simulink model "Sim_V_in"  (R2024b)
settings: Solver=VariableStepAuto  StartTime=0  StopTime=sim.t  RelTol=1e-6  AbsTol=1e-6
undefined symbols (not defined in the file or in its folder): cube, Earth, h, motor, sim, WGS84
libraries: slpidlib x3, aerolibfltsims x2, aerolibtransform2 x1, aerolibanim x1
settings Model: Creator=ben  LastModifiedBy=ben
settings DataIOCC: SaveFormat=StructureWithTime
settings OptimizationCC: BlockReduction=off  BufferReuse=off
settings DebuggingCC: SignalInfNanChecking=warning  AlgebraicLoopMsg=none  CheckMatrixSingularityMsg=warning  UnderSpecifiedDataTypeMsg=warning  UnderSpecifiedDimensionMsg=warning

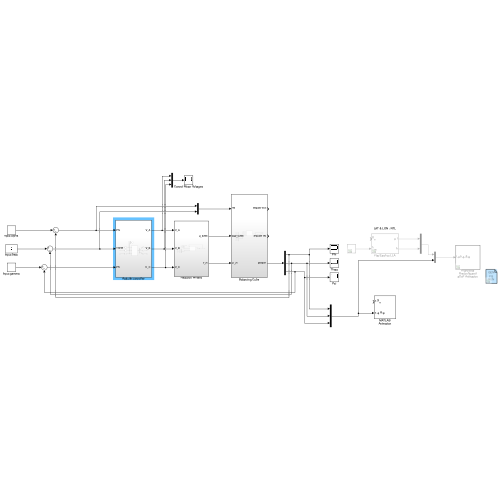
[thumbnail: Simulink's stored preview of the top-level diagram]
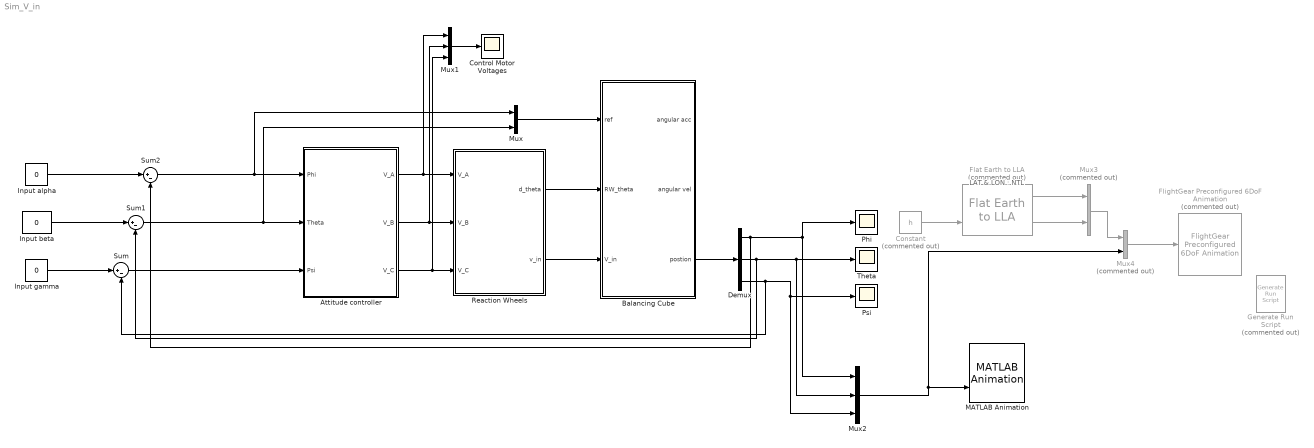
== system Sim_V_in ==
  note: LAT & LON : NTL
  Attitude controller : Subsystem
  Balancing Cube : Subsystem
  Constant : Constant  Commented=on  Value=h
  Control Motor Voltages : Scope
  Demux : Demux  Outputs=3
  Flat Earth to LLA : aerolibtransform2/Flat Earth to LLA  Commented=on  units=Metric (MKS)  ptype=Earth (WGS84)  F=1/298.257223563  R=6378137  refPosPort=off  LL0=[22 150]  psi=0
  FlightGear Preconfigured 6DoF Animation : aerolibfltsims/FlightGear Preconfigured 6DoF Animation  Commented=on  xFlightGearVersion=v2019.1  DestinationIpAddress=127.0.0.1  DestinationPort=5502  SampleTime=1/20  packetVersion=24
  Generate Run Script : aerolibfltsims/Generate Run Script  Commented=on  Architecture=Mac  dataFlow=Send  GeometryModelName=c172p  AirportId=YSSY  RunwayId=10L  InitialAltitude=7224  InitialHeading=113  OffsetDistance=4.72  OffsetAzimuth=0  InstallScenery=on  DisableShaders=on  OriginAddress=127.0.0.1  DestinationPort=5502  OriginPort=5505  LocalAddress=127.0.0.1  OutputFileName=runfg2.sh  FlightGearBaseDirectory=/Applications/FlightGear.app
  Input alpha : Constant  Value=0  SampleTime=0.1
  Input beta : Constant  Value=0  SampleTime=0.1
  Input gamma : Constant  Value=0  SampleTime=0.1
  MATLAB Animation : aerolibanim/MATLAB Animation  Tag=Matlab Animation 6 DOF  Vehicles=1  Geometries='pa24-250_orange.ac'  BoundingBoxCoordinates=[-50,50,-50,50,-50,50]  CameraOffset=[-150,0,0]  CameraViewAngle=5  SampleTime=0.01  FigurePosition=[761,103,744,778]
  Mux : Mux  Inputs=2
  Mux1 : Mux  Inputs=3
  Mux2 : Mux  Inputs=3
  Mux3 : Mux  Commented=on  Inputs=2
  Mux4 : Mux  Commented=on  Inputs=2
  Phi : Scope
  Psi : Scope
  Reaction Wheels : Subsystem
  Sum : Sum  Inputs=|+-
  Sum1 : Sum  Inputs=|+-
  Sum2 : Sum  Inputs=|+-
  Theta : Scope
  wires:
  Sum2/1 -> Mux/1, Attitude controller/1(Phi)
  Sum1/1 -> Attitude controller/2(Theta), Mux/2
  Sum/1 -> Attitude controller/3(Psi)
  Demux/1 -> Mux2/1, Phi/1, Sum2/2
  Demux/2 -> Mux2/2, Theta/1, Sum1/2
  Demux/3 -> Sum/2, Mux2/3, Psi/1
  Mux1/1 -> Control Motor Voltages/1
  Mux4/1 -> FlightGear Preconfigured 6DoF Animation/1
  Mux3/1 -> Mux4/1
  Mux2/1 -> MATLAB Animation/2, Mux4/2
  Flat Earth to LLA/2 -> Mux3/2
  Constant/1 -> Flat Earth to LLA/2
  Flat Earth to LLA/1 -> Mux3/1
  Input beta/1 -> Sum1/1
  Input gamma/1 -> Sum/1
  Reaction Wheels/2(v_in) -> Balancing Cube/3(V_in)
  Mux/1 -> Balancing Cube/1(ref)
  Balancing Cube/3(postion) -> Demux/1
  Input alpha/1 -> Sum2/1
  Attitude controller/1(V_A) -> Mux1/1, Reaction Wheels/1(V_A)
  Attitude controller/2(V_B) -> Mux1/2, Reaction Wheels/2(V_B)
  Attitude controller/3(V_C) -> Mux1/3, Reaction Wheels/3(V_C)
  Reaction Wheels/1(d_theta) -> Balancing Cube/2(RW_theta)

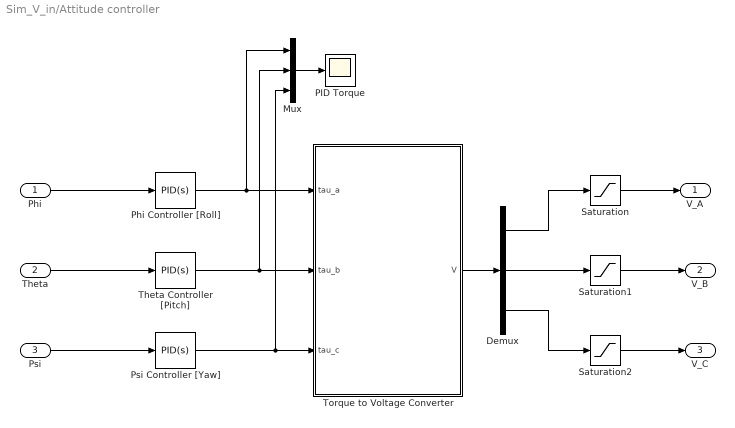
== system Sim_V_in/Attitude controller ==
  Phi : Inport
  Theta : Inport  Port=2
  Psi : Inport  Port=3
  Demux : Demux  Outputs=3
  Mux : Mux  Inputs=3
  PID Torque : Scope
  Phi Controller [Roll] : slpidlib/PID Controller  Controller=PID  Form=Parallel  TimeDomain=Continuous-time  UseExternalTs=off  SampleTime=-1  IntegratorMethod=Forward Euler  FilterMethod=Forward Euler  ControllerParametersSource=internal  P=-2.44415331656195e+90  I=-4.38149470446761e+91  UseKiTs=off  D=-3.03389489553192e+88  UseExternalDerivativeSource=off  N=5793.03682854453  UseFilter=on  TunerSelectOption=Transfer Function Based (PID Tuner App)  InitialConditionSource=internal  InitialConditionForIntegrator=0  InitialConditionForFilter=0  DifferentiatorICPrevScaledInput=0  ExternalReset=none  TrackingMode=off  Kt=1  LimitOutput=off  SatLimitsSource=internal  UpperSaturationLimit=inf  LowerSaturationLimit=-inf  LinearizeAsGain=on  AntiWindupMode=none  Kb=1  LimitIntegrator=off  UpperIntegratorSaturationLimit=inf  LowerIntegratorSaturationLimit=-inf  POutMin=[]  POutMax=[]  IOutMin=[]  IOutMax=[]  DOutMin=[]  DOutMax=[]  NOutMin=[]  NOutMax=[]  SumOutMin=[]  SumOutMax=[]  SaturationOutMin=[]  SaturationOutMax=[]  PParamMin=[]  PParamMax=[]  IParamMin=[]  IParamMax=[]  DParamMin=[]  DParamMax=[]  NParamMin=[]  NParamMax=[]  KbParamMin=[]  KbParamMax=[]  KtParamMin=[]  KtParamMax=[]  KbOutMin=[]  KbOutMax=[]  KtOutMin=[]  KtOutMax=[]  IntegratorOutMin=[]  IntegratorOutMax=[]  FilterOutMin=[]  FilterOutMax=[]  SumI1OutMin=[]  SumI1OutMax=[]  SumI2OutMin=[]  SumI2OutMax=[]  SumI3OutMin=[]  SumI3OutMax=[]  SumI4OutMin=[]  SumI4OutMax=[]  SumDOutMin=[]  SumDOutMax=[]  DifferentiatorOutMin=[]  DifferentiatorOutMax=[]  FilterDiffOutCoefMin=[]  FilterDiffOutCoefMax=[]  ReciprocalOutMin=[]  ReciprocalOutMax=[]  SumDenOutMin=[]  SumDenOutMax=[]  SumNumOutMin=[]  SumNumOutMax=[]  DivideOutMin=[]  DivideOutMax=[]  UdiffTsProdOutMin=[]  UdiffTsProdOutMax=[]  NTsProdOutMin=[]  NTsProdOutMax=[]  UintegralTsProdOutMin=[]  UintegralTsProdOutMax=[]  UngainTsProdOutMin=[]  UngainTsProdOutMax=[]  ClampingZeroOutDataTypeStr=Inherit: Inherit via back propagation  ClampingZeroOutMin=[]  ClampingZeroOutMax=[]  FilterDenConstantOutDataTypeStr=Inherit: Inherit via back propagation  FilterDenConstantOutMin=[]  FilterDenConstantOutMax=[]  PCopyOutDataTypeStr=Inherit: Inherit via back propagation  PCopyOutMin=[]  PCopyOutMax=[]  NCopyOutDataTypeStr=Inherit: Inherit via back propagation  NCopyOutMin=[]  NCopyOutMax=[]  IntegratorContinuousStateAttributes=''  IntegratorStateMustResolveToSignalObject=off  IntegratorRTWStateStorageClass=Auto  FilterContinuousStateAttributes=''  FilterStateMustResolveToSignalObject=off  FilterRTWStateStorageClass=Auto  ParallelPVariant=InternalParameters  IdealPVariant=Disabled  IVariant=InternalParameters  DVariant=InternalParameters  IntegratorVariant=Continuous  SatVariant=Disabled  AWVariant=Passthrough  PCopyVariant=Disabled  TRVariant=Disabled  FdbkBlocksVariant=Forward  IdealPFdbkVariant=Disabled  SatFdbkVariant=Disabled  DerivativeFilterVariant=ContFilter  NVariant=InternalParameters  NCopyVariant=Disabled  FilterICVariant=InternalICsFilter  IntegratorICVariant=InternalICs  ExternalResetVariant=Disabled  TRSumVariant=Passthrough  SumFdbkVariant=Disabled  SumVariant=Sum_PID  TsampFilterVariant=InternalTs  TsampNgainVariant=Passthrough  TsampIntegralVariant=Disabled_SignalSpec  ExternalSaturationOutDataTypeStr=Inherit: Same as second input  DerivativeSourceVariant=ErrorSignal  PreIntVariant=InternalPreInt
  Psi Controller [Yaw] : slpidlib/PID Controller  Controller=PID  Form=Parallel  TimeDomain=Continuous-time  UseExternalTs=off  SampleTime=-1  IntegratorMethod=Forward Euler  FilterMethod=Forward Euler  ControllerParametersSource=internal  P=-763.325878025154  I=-72.3330718489805  UseKiTs=off  D=-1552.13165448844  UseExternalDerivativeSource=off  N=226.089930864036  UseFilter=on  TunerSelectOption=Transfer Function Based (PID Tuner App)  InitialConditionSource=internal  InitialConditionForIntegrator=0  InitialConditionForFilter=0  DifferentiatorICPrevScaledInput=0  ExternalReset=none  TrackingMode=off  Kt=1  LimitOutput=off  SatLimitsSource=internal  UpperSaturationLimit=inf  LowerSaturationLimit=-inf  LinearizeAsGain=on  AntiWindupMode=none  Kb=1  LimitIntegrator=off  UpperIntegratorSaturationLimit=inf  LowerIntegratorSaturationLimit=-inf  POutMin=[]  POutMax=[]  IOutMin=[]  IOutMax=[]  DOutMin=[]  DOutMax=[]  NOutMin=[]  NOutMax=[]  SumOutMin=[]  SumOutMax=[]  SaturationOutMin=[]  SaturationOutMax=[]  PParamMin=[]  PParamMax=[]  IParamMin=[]  IParamMax=[]  DParamMin=[]  DParamMax=[]  NParamMin=[]  NParamMax=[]  KbParamMin=[]  KbParamMax=[]  KtParamMin=[]  KtParamMax=[]  KbOutMin=[]  KbOutMax=[]  KtOutMin=[]  KtOutMax=[]  IntegratorOutMin=[]  IntegratorOutMax=[]  FilterOutMin=[]  FilterOutMax=[]  SumI1OutMin=[]  SumI1OutMax=[]  SumI2OutMin=[]  SumI2OutMax=[]  SumI3OutMin=[]  SumI3OutMax=[]  SumI4OutMin=[]  SumI4OutMax=[]  SumDOutMin=[]  SumDOutMax=[]  DifferentiatorOutMin=[]  DifferentiatorOutMax=[]  FilterDiffOutCoefMin=[]  FilterDiffOutCoefMax=[]  ReciprocalOutMin=[]  ReciprocalOutMax=[]  SumDenOutMin=[]  SumDenOutMax=[]  SumNumOutMin=[]  SumNumOutMax=[]  DivideOutMin=[]  DivideOutMax=[]  UdiffTsProdOutMin=[]  UdiffTsProdOutMax=[]  NTsProdOutMin=[]  NTsProdOutMax=[]  UintegralTsProdOutMin=[]  UintegralTsProdOutMax=[]  UngainTsProdOutMin=[]  UngainTsProdOutMax=[]  ClampingZeroOutDataTypeStr=Inherit: Inherit via back propagation  ClampingZeroOutMin=[]  ClampingZeroOutMax=[]  FilterDenConstantOutDataTypeStr=Inherit: Inherit via back propagation  FilterDenConstantOutMin=[]  FilterDenConstantOutMax=[]  PCopyOutDataTypeStr=Inherit: Inherit via back propagation  PCopyOutMin=[]  PCopyOutMax=[]  NCopyOutDataTypeStr=Inherit: Inherit via back propagation  NCopyOutMin=[]  NCopyOutMax=[]  IntegratorContinuousStateAttributes=''  IntegratorStateMustResolveToSignalObject=off  IntegratorRTWStateStorageClass=Auto  FilterContinuousStateAttributes=''  FilterStateMustResolveToSignalObject=off  FilterRTWStateStorageClass=Auto  ParallelPVariant=InternalParameters  IdealPVariant=Disabled  IVariant=InternalParameters  DVariant=InternalParameters  IntegratorVariant=Continuous  SatVariant=Disabled  AWVariant=Passthrough  PCopyVariant=Disabled  TRVariant=Disabled  FdbkBlocksVariant=Forward  IdealPFdbkVariant=Disabled  SatFdbkVariant=Disabled  DerivativeFilterVariant=ContFilter  NVariant=InternalParameters  NCopyVariant=Disabled  FilterICVariant=InternalICsFilter  IntegratorICVariant=InternalICs  ExternalResetVariant=Disabled  TRSumVariant=Passthrough  SumFdbkVariant=Disabled  SumVariant=Sum_PID  TsampFilterVariant=InternalTs  TsampNgainVariant=Passthrough  TsampIntegralVariant=Disabled_SignalSpec  ExternalSaturationOutDataTypeStr=Inherit: Same as second input  DerivativeSourceVariant=ErrorSignal  PreIntVariant=InternalPreInt
  Saturation : Saturate  UpperLimit=10  LowerLimit=-10
  Saturation1 : Saturate  UpperLimit=10  LowerLimit=-10
  Saturation2 : Saturate  UpperLimit=10  LowerLimit=-10
  Theta Controller [Pitch] : slpidlib/PID Controller  Controller=PID  Form=Parallel  TimeDomain=Continuous-time  UseExternalTs=off  SampleTime=-1  IntegratorMethod=Forward Euler  FilterMethod=Forward Euler  ControllerParametersSource=internal  P=-8.13203404050408e+20  I=-3.59982541336858e+22  UseKiTs=off  D=-4.51084621020332e+18  UseExternalDerivativeSource=off  N=4975.57673271944  UseFilter=on  TunerSelectOption=Transfer Function Based (PID Tuner App)  InitialConditionSource=internal  InitialConditionForIntegrator=0  InitialConditionForFilter=0  DifferentiatorICPrevScaledInput=0  ExternalReset=none  TrackingMode=off  Kt=1  LimitOutput=off  SatLimitsSource=internal  UpperSaturationLimit=inf  LowerSaturationLimit=-inf  LinearizeAsGain=on  AntiWindupMode=none  Kb=1  LimitIntegrator=off  UpperIntegratorSaturationLimit=inf  LowerIntegratorSaturationLimit=-inf  POutMin=[]  POutMax=[]  IOutMin=[]  IOutMax=[]  DOutMin=[]  DOutMax=[]  NOutMin=[]  NOutMax=[]  SumOutMin=[]  SumOutMax=[]  SaturationOutMin=[]  SaturationOutMax=[]  PParamMin=[]  PParamMax=[]  IParamMin=[]  IParamMax=[]  DParamMin=[]  DParamMax=[]  NParamMin=[]  NParamMax=[]  KbParamMin=[]  KbParamMax=[]  KtParamMin=[]  KtParamMax=[]  KbOutMin=[]  KbOutMax=[]  KtOutMin=[]  KtOutMax=[]  IntegratorOutMin=[]  IntegratorOutMax=[]  FilterOutMin=[]  FilterOutMax=[]  SumI1OutMin=[]  SumI1OutMax=[]  SumI2OutMin=[]  SumI2OutMax=[]  SumI3OutMin=[]  SumI3OutMax=[]  SumI4OutMin=[]  SumI4OutMax=[]  SumDOutMin=[]  SumDOutMax=[]  DifferentiatorOutMin=[]  DifferentiatorOutMax=[]  FilterDiffOutCoefMin=[]  FilterDiffOutCoefMax=[]  ReciprocalOutMin=[]  ReciprocalOutMax=[]  SumDenOutMin=[]  SumDenOutMax=[]  SumNumOutMin=[]  SumNumOutMax=[]  DivideOutMin=[]  DivideOutMax=[]  UdiffTsProdOutMin=[]  UdiffTsProdOutMax=[]  NTsProdOutMin=[]  NTsProdOutMax=[]  UintegralTsProdOutMin=[]  UintegralTsProdOutMax=[]  UngainTsProdOutMin=[]  UngainTsProdOutMax=[]  ClampingZeroOutDataTypeStr=Inherit: Inherit via back propagation  ClampingZeroOutMin=[]  ClampingZeroOutMax=[]  FilterDenConstantOutDataTypeStr=Inherit: Inherit via back propagation  FilterDenConstantOutMin=[]  FilterDenConstantOutMax=[]  PCopyOutDataTypeStr=Inherit: Inherit via back propagation  PCopyOutMin=[]  PCopyOutMax=[]  NCopyOutDataTypeStr=Inherit: Inherit via back propagation  NCopyOutMin=[]  NCopyOutMax=[]  IntegratorContinuousStateAttributes=''  IntegratorStateMustResolveToSignalObject=off  IntegratorRTWStateStorageClass=Auto  FilterContinuousStateAttributes=''  FilterStateMustResolveToSignalObject=off  FilterRTWStateStorageClass=Auto  ParallelPVariant=InternalParameters  IdealPVariant=Disabled  IVariant=InternalParameters  DVariant=InternalParameters  IntegratorVariant=Continuous  SatVariant=Disabled  AWVariant=Passthrough  PCopyVariant=Disabled  TRVariant=Disabled  FdbkBlocksVariant=Forward  IdealPFdbkVariant=Disabled  SatFdbkVariant=Disabled  DerivativeFilterVariant=ContFilter  NVariant=InternalParameters  NCopyVariant=Disabled  FilterICVariant=InternalICsFilter  IntegratorICVariant=InternalICs  ExternalResetVariant=Disabled  TRSumVariant=Passthrough  SumFdbkVariant=Disabled  SumVariant=Sum_PID  TsampFilterVariant=InternalTs  TsampNgainVariant=Passthrough  TsampIntegralVariant=Disabled_SignalSpec  ExternalSaturationOutDataTypeStr=Inherit: Same as second input  DerivativeSourceVariant=ErrorSignal  PreIntVariant=InternalPreInt
  Torque to Voltage Converter : MATLAB Function  TreatAsAtomicUnit=on
  V_A : Outport
  V_B : Outport  Port=2
  V_C : Outport  Port=3
  wires:
  Phi/1 -> Phi Controller [Roll]/1
  Theta/1 -> Theta Controller [Pitch]/1
  Psi/1 -> Psi Controller [Yaw]/1
  Theta Controller [Pitch]/1 -> Mux/2, Torque to Voltage Converter/2(tau_b)
  Phi Controller [Roll]/1 -> Mux/1, Torque to Voltage Converter/1(tau_a)
  Psi Controller [Yaw]/1 -> Mux/3, Torque to Voltage Converter/3(tau_c)
  Demux/2 -> Saturation1/1
  Demux/3 -> Saturation2/1
  Mux/1 -> PID Torque/1
  Saturation/1 -> V_A/1
  Saturation1/1 -> V_B/1
  Saturation2/1 -> V_C/1
  Torque to Voltage Converter/1(V) -> Demux/1
  Demux/1 -> Saturation/1

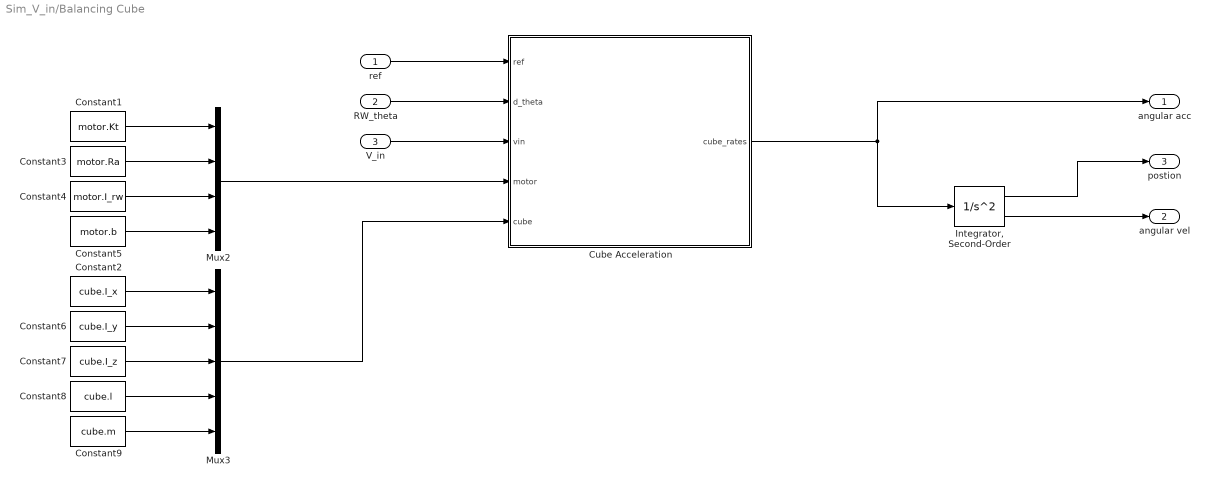
== system Sim_V_in/Balancing Cube ==
  ref : Inport
  RW_theta : Inport  Port=2
  V_in : Inport  Port=3
  Constant1 : Constant  Value=motor.Kt
  Constant2 : Constant  Value=cube.I_x
  Constant3 : Constant  Value=motor.Ra
  Constant4 : Constant  Value=motor.I_rw
  Constant5 : Constant  Value=motor.b
  Constant6 : Constant  Value=cube.I_y
  Constant7 : Constant  Value=cube.I_z
  Constant8 : Constant  Value=cube.l
  Constant9 : Constant  Value=cube.m
  Cube Acceleration : MATLAB Function  TreatAsAtomicUnit=on
  "Integrator, Second-Order" : SecondOrderIntegrator  ICX=sim.cube_ic_pos  ICDXDT=sim.cube_ic_vel
  Mux2 : Mux
  Mux3 : Mux  Inputs=5
  angular acc : Outport
  angular vel : Outport  Port=2
  postion : Outport  Port=3
  wires:
  ref/1 -> Cube Acceleration/1(ref)
  RW_theta/1 -> Cube Acceleration/2(d_theta)
  V_in/1 -> Cube Acceleration/3(vin)
  Constant5/1 -> Mux2/4
  Constant3/1 -> Mux2/2
  Constant4/1 -> Mux2/3
  Constant9/1 -> Mux3/5
  Constant7/1 -> Mux3/3
  Constant1/1 -> Mux2/1
  Constant6/1 -> Mux3/2
  Constant2/1 -> Mux3/1
  Constant8/1 -> Mux3/4
  Mux2/1 -> Cube Acceleration/4(motor)
  Mux3/1 -> Cube Acceleration/5(cube)
  Cube Acceleration/1(cube_rates) -> angular acc/1, "Integrator, Second-Order"/1
  "Integrator, Second-Order"/2 -> angular vel/1
  "Integrator, Second-Order"/1 -> postion/1

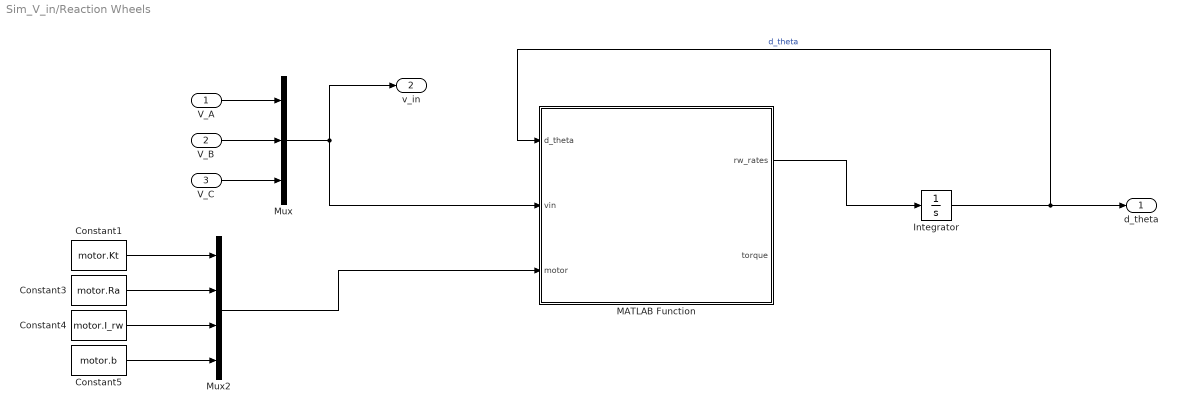
== system Sim_V_in/Reaction Wheels ==
  V_A : Inport
  V_B : Inport  Port=2
  V_C : Inport  Port=3
  Constant1 : Constant  Value=motor.Kt
  Constant3 : Constant  Value=motor.Ra
  Constant4 : Constant  Value=motor.I_rw
  Constant5 : Constant  Value=motor.b
  Integrator : Integrator  InitialCondition=sim.rw_ic
  MATLAB Function : MATLAB Function  TreatAsAtomicUnit=on
  Mux : Mux  Inputs=3
  Mux2 : Mux
  d_theta : Outport
  v_in : Outport  Port=2
  wires:
  Integrator/1 -> MATLAB Function/1(d_theta), d_theta/1  "d_theta"
  V_A/1 -> Mux/1
  V_B/1 -> Mux/2
  V_C/1 -> Mux/3
  Mux/1 -> MATLAB Function/2(vin), v_in/1
  Mux2/1 -> MATLAB Function/3(motor)
  Constant1/1 -> Mux2/1
  Constant3/1 -> Mux2/2
  Constant5/1 -> Mux2/4
  Constant4/1 -> Mux2/3
  MATLAB Function/1(rw_rates) -> Integrator/1

== matlab function Sim_V_in/Reaction Wheels/MATLAB Function ==
  data: d_theta input; vin input; motor input; rw_rates output size=[3 ,1]; torque output
function [rw_rates,torque]  = rw_acc(d_theta, vin, motor)
    %% Extract parameters
    Kt = motor(1);
    Ra = motor(2);
    I_w = motor(3);
    b = motor(4);

    d_theta_A = d_theta(1);
    d_theta_B = d_theta(2);
    d_theta_C = d_theta(3);

    V_A = vin(1);
    V_B = vin(2);
    V_C = vin(3);

    R_y = [cos(-35.3*pi/180) 0 sin(-35.3*pi/180); 0 1 0; -sin(-35.3*pi/180) 0 cos(-35.3*pi/180)];
    R_x = [1 0 0; 0 cos(45*pi/180) -sin(45*pi/180); 0 sin(45*pi/180) cos(45*pi/180)];
    
    T_bf = R_y * R_x;

    %% Caclulate Angular Rates of Reaction Wheels
    % Simplified model
    dd_theta_A = ((Kt/Ra) * (V_A - Kt * d_theta_A))/I_w;
    dd_theta_B = ((Kt/Ra) * (V_B - Kt * d_theta_B))/I_w;
    dd_theta_C = ((Kt/Ra) * (V_C - Kt * d_theta_C))/I_w;

    % Complex Model
    % dd_theta_A = ((Kt/Ra) * (V_A - Kt * d_theta_A) - b * d_theta_A)/I_w;
    % dd_theta_B = ((Kt/Ra) * (V_B - Kt * d_theta_B) - b * d_theta_B)/I_w;
    % dd_theta_C = ((Kt/Ra) * (V_C - Kt * d_theta_C) - b * d_theta_C)/I_w;

    rw_rates = [dd_theta_A; dd_theta_B; dd_theta_C];

    tau_x = (Kt/Ra) * (V_A - Kt * d_theta_A) - b * d_theta_A;
    tau_y = (Kt/Ra) * (V_B - Kt * d_theta_B) - b * d_theta_B;
    tau_z = (Kt/Ra) * (V_C - Kt * d_theta_C) - b * d_theta_C;

    torque = [tau_x; tau_y; tau_z];

end

== matlab function Sim_V_in/Attitude controller/Torque to Voltage Converter ==
  data: tau_a input; V output; tau_b input; tau_c input
function V = tau_to_V(tau_a, tau_b, tau_c)
    % V_A, V_B, V_C]
    % V_A = tau_a/2 + tau_b/2;
    % V_B = tau_b + ((tau_g - tau_a/2)- 3*tau_b/2)/3;
    % V_C = ((tau_g - tau_a/2)- 3*tau_b/2)/3;

    
    % From Geometric Configuration
    m = [2 -1 -1;0 1 -1; 1 1 1];


    t = [tau_a; tau_b; tau_c];

    V = t\(m);

== matlab function Sim_V_in/Balancing Cube/Cube Acceleration ==
  data: ref input; cube_rates output size=[3,1]; d_theta input; vin input; motor input; cube input
function cube_rates = cube_acc(ref, d_theta, vin, motor, cube) 
    %% Extract parameters
    alpha = ref(1);
    beta = ref(2);

    Kt = motor(1);
    Ra = motor(2);
    I_w = motor(3);
    b = motor(4);

    I_x = cube(1);
    I_y = cube(2);
    I_z = cube(3);
    l = cube(4);
    m = cube(5);

    g = 9.81;  % Gravitational constant

    d_theta_A = d_theta(1);
    d_theta_B = d_theta(2);
    d_theta_C = d_theta(3);

    V_A = vin(1);
    V_B = vin(2);
    V_C = vin(3);

    
    %% Caclulate Angular Rates of Reaction Wheels
    % Simplified model
    dd_alpha = (m*g*l*sin(alpha)*cos(beta) - (sqrt(6)/6)*(Kt/Ra)*((-2*V_A + V_B + V_C) - Kt*(2*d_theta_A - d_theta_B - d_theta_C))) / (I_y - I_w);
    dd_beta = (-m*g*l*sin(beta)*cos(alpha) - (sqrt(2)/2)*(Kt/Ra)*((V_B - V_C) -Kt*(d_theta_B - d_theta_C))) /(I_x - I_w);
    dd_gamma =  ((sqrt(3)/3)*(Kt/Ra)*((V_A + V_B + V_C) - Kt*(d_theta_A + d_theta_B + d_theta_C))) / (I_z - I_w);
    
    % Complex Model
    % dd_alpha = (m*g*l*sin(alpha)*cos(beta) - (sqrt(6)/6)*(Kt/Ra)*((-2*V_A + V_B + V_C) - Kt*(2*d_theta_A - d_theta_B - d_theta_C)- b*(2*d_theta_A - d_theta_B - d_theta_C))) / (I_y - I_w);
    % dd_beta = (-m*g*l*sin(beta)*cos(alpha) - (sqrt(2)/2)*(Kt/Ra)*((V_B - V_C) -Kt*(d_theta_B - d_theta_C)- b*(d_theta_B - d_theta_C))) /(I_x - I_w);
    % dd_gamma =  ((sqrt(3)/3)*(Kt/Ra)*((V_A + V_B + V_C) - Kt*(d_theta_A + d_theta_B + d_theta_C)- b*(d_theta_A + d_theta_B + d_theta_C))) / (I_z - I_w);

    cube_rates = [dd_alpha; dd_beta; dd_gamma];
    % cube_rates = T_bf *[dd_alpha; dd_beta; dd_gamma];
end
